simulink library "SG_library"  (R2022b)
settings: Solver=VariableStepAuto  StartTime=0.0  StopTime=10.0  RelTol=1e-3
undefined symbols (not defined in the file or in its folder): a, b, c, ctrl_limit, dfilt, GeneratorType, IO324, IO324_FPGA, IO324_src, IO334, IO334_FPGA, IO334_src, IO397, IO397_FPGA, IO397_src, repelem
libraries: speedgoatlib_hdlCoder_IO3xx x44, $bdroot x14, slrealtimeutilitieslib x9, simulink x8, hdlsllib x6, dsparch4 x2
(part 1 of 3)
settings Model: Creator=mavolery  LastModifiedBy=mavolery

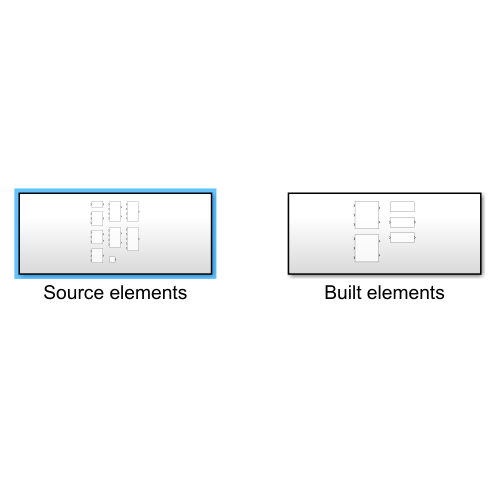
[thumbnail: Simulink's stored preview of the top-level diagram]
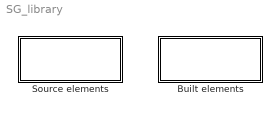
== system SG_library ==
  Built elements : Subsystem
  Source elements : Subsystem

== system SG_library/Built elements ==
  IO324_IO : Subsystem  mask(IO334 IO){ts=-1, adcGain=5.12V, dacGain=5.0V}
      mask prompts: ts "Filters sampling time"; adcGain "ADC range (all channels)"; dacGain "DAC range (all channels)"
      mask help: Links the 16 first physical analog inputs/outputs to the CPU part of the speedgoat.
      mask TypeOptions ts: IO324_SOS/ts
      mask TypeOptions adcGain: IO324_SOS/adcGain
      mask TypeOptions dacGain: IO324_SOS/dacGain
  IO324_SOS : Subsystem  mask(IO334_SOS){sos1=[0 0 0 1 0 0;0 0 0 1 0 0;0 0 0 1 0 0;0 0 0 1 0 0], sos2=[0 0 0 1 0 0;0 0 0 1 0 0;0 0 0 1 0 0;0 0 0 1 0 0], ctrl_limit=-1, ts=-1, channel_in=[1 2], channel_out=1, adcGain=5.12V, dacGain=5.0V}
      mask prompts: sos1 "SOS matrix AI1 -> AO1"; sos2 "SOS matrix AI2 -> AO1"; ctrl_limit "Control output limit [V]"; ts "Filters sampling time"; channel_in "Filter input channels (1-16, 0 for GND)"; channel_out "Filter output channel (1-8)"; adcGain "ADC range (all channels)"; dacGain "DAC range (all channels)"
      mask help: Implements a discrete fixed-point filter by second order sections cascade. SOS matrices are given by tf2sos or zp2sos.
      mask TypeOptions adcGain: IO324_FPGA/adcGain_1 | IO324_FPGA/adcGain_10 | IO324_FPGA/adcGain_11 | IO324_FPGA/adcGain_12 | IO324_FPGA/adcGain_13 | IO324_FPGA/adcGain_14 | IO324_FPGA/adcGain_15 | IO324_FPGA/adcGain_16 | IO324_FPGA/adcGain_17 | IO324_FPGA/adcGain_18 | IO324_FPGA/adcGain_19 | IO324_FPGA/adcGain_2 | IO324_FPGA/adcGain_20 | IO324_FPGA/adcGain_21 | IO324_FPGA/adcGain_22 | IO324_FPGA/adcGain_23 | IO324_FPGA/adcGain_24 | IO324_FPGA/adcGain_25 | IO324_FPGA/adcGain_26 | IO324_FPGA/adcGain_27 | IO324_FPGA/adcGain_28 | IO324_FPGA/adcGain_29 | IO324_FPGA/adcGain_3 | IO324_FPGA/adcGain_30 | IO324_FPGA/adcGain_31 | IO324_FPGA/adcGain_32 | IO324_FPGA/adcGain_4 | IO324_FPGA/adcGain_5 | IO324_FPGA/adcGain_6 | IO324_FPGA/adcGain_7 | IO324_FPGA/adcGain_8 | IO324_FPGA/adcGain_9
      mask TypeOptions dacGain: IO324_FPGA/dacGain_1 | IO324_FPGA/dacGain_2 | IO324_FPGA/dacGain_3 | IO324_FPGA/dacGain_4 | IO324_FPGA/dacGain_5 | IO324_FPGA/dacGain_6 | IO324_FPGA/dacGain_7 | IO324_FPGA/dacGain_8
  IO334_IO : Subsystem  mask(IO334 IO){ts=-1, span=Auto (same as ADC)}
      mask prompts: ts "Sampling time (ADC)"; span "DAC Voltage Range:"
      mask help: Links the 16 first physical analog inputs/outputs to the CPU part of the speedgoat.
      mask TypeOptions ts: IO334_SOS/ts
      mask TypeOptions span: IO334_SOS/span
  IO334_SOS : Subsystem  mask(IO334_SOS){sos1=[0 0 0 1 0 0;0 0 0 1 0 0;0 0 0 1 0 0;0 0 0 1 0 0], sos2=[0 0 0 1 0 0;0 0 0 1 0 0;0 0 0 1 0 0;0 0 0 1 0 0], limit_ctrl=-1, channel_in=[1 2], channel_out=1, ts=-1, span=Auto (same as ADC)}
      mask prompts: sos1 "SOS matrix AI1 -> AO1"; sos2 "SOS matrix AI2 -> AO1"; limit_ctrl "Control output limit [V]"; channel_in "Filter input channels (1-16, 0 for GND)"; channel_out "filtouer output channel (1-16)"; ts "Sampling time (ADC)"; span "DAC Voltage Range:"
      mask help: Implements a discrete fixed-point filter by second order sections cascade. SOS matrices are given by tf2sos or zp2sos.
      mask TypeOptions span: IO334_FPGA/OutputRange
  IO397_IO : Subsystem  mask(IO397 IO){ts=-1, range1=+-10 V, range2=+-10 V, range3=+-10 V, range4=+-10 V, span=+-10 V}
      mask prompts: ts "Sampling time (ADC)"; range1 "Range ADC Channel 1"; range2 "Range ADC Channel 2"; range3 "Range ADC Channel 3"; range4 "Range ADC Channel 4"; span "DAC Voltage Span:"
      mask help: Links the four first physical analog inputs/outputs to the CPU part of the speedgoat.
      mask TypeOptions ts: IO397_SOS/ts
      mask TypeOptions range1: IO397_SOS/range1
      mask TypeOptions range2: IO397_SOS/range2
      mask TypeOptions range3: IO397_SOS/range3
      mask TypeOptions range4: IO397_SOS/range4
      mask TypeOptions span: IO397_SOS/span
      mask DialogControl AnalogInput Prompt: Analog Inputs
      mask DialogControl AnalogOutput Prompt: Analog Output
  IO397_SOS : Subsystem  mask(IO397_SOS){sos1=[1 0 0 1 0 0;1 0 0 1 0 0;1 0 0 1 0 0;1 0 0 1 0 0], sos2=[0 0 0 1 0 0;0 0 0 1 0 0;0 0 0 1 0 0;0 0 0 1 0 0], limit_ctrl=-1, ts=-1, channel_in=[1,2], channel_out=1, range1=+-10 V, range2=+-10 V, range3=+-10 V, range4=+-10 V, span=+-10 V}
      mask prompts: sos1 "SOS matrix AI1 -> AO1"; sos2 "SOS matrix AI2 -> AO1"; limit_ctrl "Control output limit [V]"; ts "Sampling time (ADC)"; channel_in "Filter input channels (1-4, 0 for gnd)"; channel_out "Filter output channel (1-4)"; range1 "Range ADC Channel 1"; range2 "Range ADC Channel 2"; range3 "Range ADC Channel 3"; range4 "Range ADC Channel 4"; span "DAC Voltage Span:"
      mask help: Implements a discrete fixed-point filter by second order sections cascade. SOS matrices are given by tf2sos or zp2sos.
      mask init:
      | assert(all(range1 ~= [1 4 5]), 'ADC1 range must be symetric');
      | assert(all(range2 ~= [1 4 5]), 'ADC2 range must be symetric');
      | assert(all(span ~= [1 2]), 'DAC span must be symetric');
      mask TypeOptions range1: IO397_FPGA/range1
      mask TypeOptions range2: IO397_FPGA/range2
      mask TypeOptions range3: IO397_FPGA/range3
      mask TypeOptions range4: IO397_FPGA/range4
      mask TypeOptions span: IO397_FPGA/span
      mask DialogControl AnalogInput Prompt: Analog Inputs
      mask DialogControl AnalogOutput Prompt: Analog Output
  private : Subsystem

== system SG_library/Source elements ==
  ADC trigger : Subsystem  mask(AI trigger){}
      mask help: Creates a boolean pulse every given cylces. It can be use for ADC acquisition
  Discrete SOS section DFI serial : Subsystem  mask(Discrete fixed-point SOS section){idx=1, OutDataTypeStr=fixdt(1,80,52)}
      mask prompts: idx "Index"; OutDataTypeStr "Accumulator datatype"
      mask help: This is a fixed-point implementation of a biquad filter. Specify the sos [N/2, 6] matrix e.g. given by tf2sos or zpk2sos functions. The first denominator coefficient must always be equal to 1. Index (1 - N/2) parameter specifies which section of the filter is implemented.
      mask TypeOptions OutDataTypeStr: Signal Specification/OutDataTypeStr
  Discrete SOS serial : Subsystem  mask(Discrete fixed-point second order sections filter){OutDataTypeStr=fixdt(1,80,52)}
      mask prompts: OutDataTypeStr "Accumulator datatype"
      mask help: This is a SOS implemetation of order 8 (4 sections). Specify the sos [n/2, 6] matrix e.g. given by tf2sos function. The first denominator coefficient must always be equal to 1.
      mask TypeOptions OutDataTypeStr:
      | Discrete SOS
      | section DFI serial/OutDataTypeStr
  Generator : Subsystem  mask(Generator){duration=10, rms=1, f1=50, f2=500, gen_type=GeneratorType.rand_white, ts=-1}
      mask prompts: duration "Duration [s]"; rms "RMS value"; f1 "Start frequency [Hz] (sweep only)"; f2 "Stop frequency [Hz] (sweep only)"; gen_type "Type (GeneratorType)"; ts "Sampling time [s]"
      mask help: Runs different types of generators for a given duration. Generator can be triggered, canceled and manually enabled.
  Linear Chirp : Subsystem  mask{f1=10, f2=50, t_sweep=2.64, ts=-1}
      mask prompts: f1 "Start frequency"; f2 "End frequency"; t_sweep "Sweep time"; ts "Sample time"
  Logarithmic Chirp : Subsystem  mask{f1=10, f2=50, t_sweep=2.64, ts=-1}
      mask prompts: f1 "Start frequency"; f2 "End frequency"; t_sweep "Sweep time"; ts "Sample time"
  Random source : Subsystem  mask(Random source){mean=0, stdev=1, seed=0, SampleTime=0.0001}
      mask prompts: stdev "Standard deviation"; SampleTime "Sample time"
      mask help: Creates some random signal, limited in frequency at Fs/4
  SOS filter : Subsystem  mask(SOS filter){sos1=[0 0 0 1 0 0;0 0 0 1 0 0;0 0 0 1 0 0;0 0 0 1 0 0], sos2=[0 0 0 1 0 0;0 0 0 1 0 0;0 0 0 1 0 0;0 0 0 1 0 0], limit_ctrl=10, ts=-1}
      mask prompts: sos1 "SOS matrix AI1 -> AO1"; sos2 "SOS matrix AI2 -> AO1"; limit_ctrl "Control output limit [V]"; ts "Filter sampling time [s]"
      mask help: Implements a discrete fixed-point filter by second order sections cascade. SOS matrices are given by tf2sos or zp2sos.
  Triggered Pulse : Subsystem  mask(Triggered Pulse){}
      mask help: Generates a single pulse of N samples length

== system SG_library/Built elements/IO324_IO ==
  AO : Inport
  Constant : Constant  Value=false  SampleTime=-1
  Constant1 : Constant  Value=false  SampleTime=-1
  IO324_SOS : $bdroot/Built elements/IO324_SOS  sos1=[0 0 0 1 0 0;0 0 0 1 0 0;0 0 0 1 0 0;0 0 0 1 0 0]  sos2=[0 0 0 1 0 0;0 0 0 1 0 0;0 0 0 1 0 0;0 0 0 1 0 0]  ctrl_limit=-1  ts=ts  channel_in=[1 2]  channel_out=1  adcGain=5.12V  dacGain=5.0V
      settings: LibrarySourceBlock=libpanache/IO324_SOS
  Rate Transition : RateTransition  OutPortSampleTime=ts
  Terminator : Terminator
  Terminator1 : Terminator
  AI : Outport  VectorParamsAs1DForOutWhenUnconnected=off
  wires:
  Constant/1 -> IO324_SOS/2
  AO/1 -> IO324_SOS/1
  IO324_SOS/1 -> Rate Transition/1
  Rate Transition/1 -> AI/1
  IO324_SOS/2 -> Terminator/1
  Constant1/1 -> IO324_SOS/3
  IO324_SOS/3 -> Terminator1/1

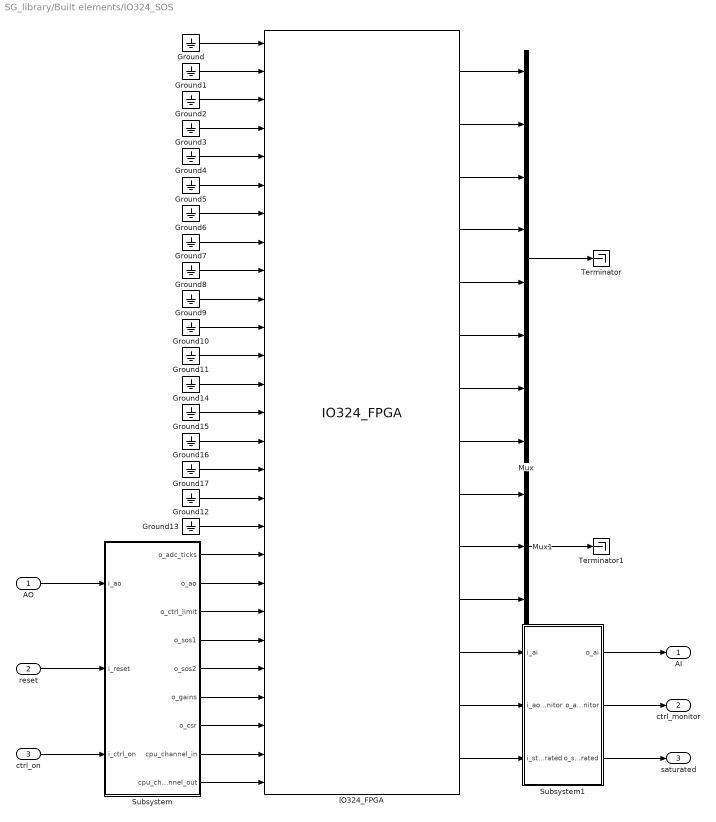
== system SG_library/Built elements/IO324_SOS ==
  AO : Inport  PortDimensions=8
  reset : Inport  Port=2  OutDataTypeStr=boolean  PortDimensions=1
  ctrl_on : Inport  Port=3  OutDataTypeStr=boolean  PortDimensions=1
  Ground{,1..17} (18 alike) : Ground
  IO324_FPGA : $bdroot/Built elements/private/IO324_FPGA  module_id=1  slot=-1  ts=-1  adcGain_1=5.12V  adcActiv_1=on  adcDiffSelect_1=off  adcGain_2=5.12V  adcActiv_2=on  adcDiffSelect_2=off  adcGain_3=5.12V  adcActiv_3=off  adcDiffSelect_3=off  adcGain_4=5.12V  adcActiv_4=off  adcDiffSelect_4=off  adcGain_5=5.12V  adcActiv_5=off  adcDiffSelect_5=off  adcGain_6=5.12V  adcActiv_6=off  adcDiffSelect_6=off  adcGain_7=5.12V  adcActiv_7=off  adcDiffSelect_7=off  adcGain_8=5.12V  adcActiv_8=off  adcDiffSelect_8=off  adcGain_9=5.12V  adcActiv_9=on  adcDiffSelect_9=off  adcGain_10=5.12V  adcActiv_10=on  adcDiffSelect_10=off  adcGain_11=5.12V  adcActiv_11=off  adcDiffSelect_11=off  adcGain_12=5.12V  adcActiv_12=off  adcDiffSelect_12=off  adcGain_13=5.12V  adcActiv_13=off  adcDiffSelect_13=off  adcGain_14=5.12V  adcActiv_14=off  adcDiffSelect_14=off  adcGain_15=5.12V  adcActiv_15=off  adcDiffSelect_15=off  adcGain_16=5.12V  adcActiv_16=off  adcDiffSelect_16=off  adcGain_17=5.12V  adcActiv_17=on  adcDiffSelect_17=off  adcGain_18=5.12V  adcActiv_18=on  adcDiffSelect_18=off  adcGain_19=5.12V  adcActiv_19=off  adcDiffSelect_19=off  adcGain_20=5.12V  adcActiv_20=off  adcDiffSelect_20=off  adcGain_21=5.12V  adcActiv_21=off  adcDiffSelect_21=off  adcGain_22=5.12V  adcActiv_22=off  adcDiffSelect_22=off  adcGain_23=5.12V  adcActiv_23=off  adcDiffSelect_23=off  adcGain_24=5.12V  adcActiv_24=off  adcDiffSelect_24=off  adcGain_25=5.12V  adcActiv_25=on  adcDiffSelect_25=off  adcGain_26=5.12V  adcActiv_26=on  adcDiffSelect_26=off  adcGain_27=5.12V  adcActiv_27=off  adcDiffSelect_27=off  adcGain_28=5.12V  adcActiv_28=off  adcDiffSelect_28=off  adcGain_29=5.12V  adcActiv_29=off  adcDiffSelect_29=off  adcGain_30=5.12V  adcActiv_30=off  adcDiffSelect_30=off  adcGain_31=5.12V  adcActiv_31=off  adcDiffSelect_31=off  adcGain_32=5.12V  adcActiv_32=off  adcDiffSelect_32=off  dacGain_1=5.0V  dacActiv_1=on  dacGain_2=5.0V  dacActiv_2=on  dacGain_3=5.0V  dacActiv_3=on  dacGain_4=5.0V  dacActiv_4=on  dacGain_5=5.0V  dacActiv_5=on  dacGain_6=5.0V  dacActiv_6=on  dacGain_7=5.0V  dacActiv_7=on  dacGain_8=5.0V  dacActiv_8=on  fpga_sync_mode=on  reset_mode=on  reset_mode_stop=on  FpgaFreq=100
      settings: LibrarySourceBlock=libpanache/private/IO324_FPGA
  Mux : Mux  Inputs=8
  Mux1 : Mux  Inputs=3
  Subsystem : Subsystem
  Subsystem1 : Subsystem
  Terminator : Terminator
  Terminator1 : Terminator
  AI : Outport  VectorParamsAs1DForOutWhenUnconnected=off
  ctrl_monitor : Outport  Port=2  VectorParamsAs1DForOutWhenUnconnected=off
  saturated : Outport  Port=3
  wires:
  Ground/1 -> IO324_FPGA/1
  Ground1/1 -> IO324_FPGA/2
  Ground2/1 -> IO324_FPGA/3
  Ground3/1 -> IO324_FPGA/4
  Ground4/1 -> IO324_FPGA/5
  Ground7/1 -> IO324_FPGA/8
  Ground6/1 -> IO324_FPGA/7
  Ground5/1 -> IO324_FPGA/6
  Ground9/1 -> IO324_FPGA/10
  Ground10/1 -> IO324_FPGA/11
  Ground8/1 -> IO324_FPGA/9
  Ground11/1 -> IO324_FPGA/12
  AO/1 -> Subsystem/1(i_ao)
  ctrl_on/1 -> Subsystem/3(i_ctrl_on)
  reset/1 -> Subsystem/2(i_reset)
  Subsystem1/1(o_ai) -> AI/1
  Subsystem1/2(o_ao_monitor) -> ctrl_monitor/1
  IO324_FPGA/12 -> Subsystem1/1(i_ai)
  IO324_FPGA/13 -> Subsystem1/2(i_ao_monitor)
  Subsystem/7(o_csr) -> IO324_FPGA/25
  Subsystem/2(o_ao) -> IO324_FPGA/20
  Subsystem/3(o_ctrl_limit) -> IO324_FPGA/21
  Subsystem/4(o_sos1) -> IO324_FPGA/22
  Subsystem/5(o_sos2) -> IO324_FPGA/23
  Subsystem/6(o_gains) -> IO324_FPGA/24
  Subsystem/1(o_adc_ticks) -> IO324_FPGA/19
  Ground16/1 -> IO324_FPGA/15
  Ground12/1 -> IO324_FPGA/17
  Ground17/1 -> IO324_FPGA/16
  Ground15/1 -> IO324_FPGA/14
  Ground14/1 -> IO324_FPGA/13
  Ground13/1 -> IO324_FPGA/18
  IO324_FPGA/1 -> Mux/1
  IO324_FPGA/2 -> Mux/2
  IO324_FPGA/3 -> Mux/3
  IO324_FPGA/4 -> Mux/4
  IO324_FPGA/5 -> Mux/5
  IO324_FPGA/6 -> Mux/6
  IO324_FPGA/7 -> Mux/7
  IO324_FPGA/8 -> Mux/8
  Mux/1 -> Terminator/1
  IO324_FPGA/9 -> Mux1/1
  IO324_FPGA/10 -> Mux1/2
  IO324_FPGA/11 -> Mux1/3
  IO324_FPGA/14 -> Subsystem1/3(i_staurated)
  Subsystem1/3(o_saturated) -> saturated/1
  Subsystem/8(cpu_channel_in) -> IO324_FPGA/26
  Subsystem/9(cpu_channel_out) -> IO324_FPGA/27
  Mux1/1 -> Terminator1/1

== system SG_library/Built elements/IO334_IO ==
  AO : Inport
  Constant : Constant  Value=false  SampleTime=-1
  IO334_SOS : $bdroot/Built elements/IO334_SOS  sos1=[0 0 0 1 0 0;0 0 0 1 0 0;0 0 0 1 0 0;0 0 0 1 0 0]  sos2=[0 0 0 1 0 0;0 0 0 1 0 0;0 0 0 1 0 0;0 0 0 1 0 0]  limit_ctrl=-1  channel_in=[1 2]  channel_out=1  ts=ts  span=Auto (same as ADC)
      settings: LibrarySourceBlock=SG_library_TRASH/Built elements/IO334_SOS
  Rate Transition : RateTransition  OutPortSampleTime=ts
  Terminator : Terminator
  Terminator1 : Terminator
  AI : Outport  VectorParamsAs1DForOutWhenUnconnected=off
  wires:
  Constant/1 -> IO334_SOS/3, IO334_SOS/2
  AO/1 -> IO334_SOS/1
  IO334_SOS/1 -> Rate Transition/1
  Rate Transition/1 -> AI/1
  IO334_SOS/2 -> Terminator/1
  IO334_SOS/3 -> Terminator1/1

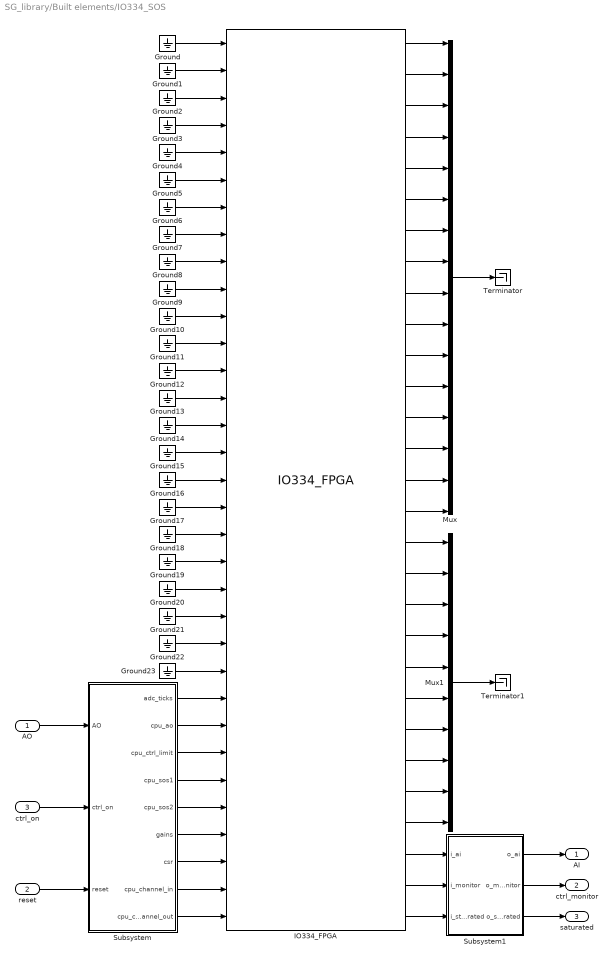
== system SG_library/Built elements/IO334_SOS ==
  AO : Inport
  reset : Inport  Port=2
  ctrl_on : Inport  Port=3
  Ground{,1..23} (24 alike) : Ground
  IO334_FPGA : $bdroot/Built elements/private/IO334_FPGA  module_id=1  slot=-1  ts=-1  OutputRange=Auto (same as ADC)  fpga_sync_mode=on  reset_mode=on  reset_mode_stop=on  FpgaFreq=100
      settings: LibrarySourceBlock=SG_library_TRASH/Built elements/private/IO334_FPGA
  Mux : Mux  Inputs=16
  Mux1 : Mux  Inputs=10
  Subsystem : Subsystem
  Subsystem1 : Subsystem
  Terminator : Terminator
  Terminator1 : Terminator
  AI : Outport  VectorParamsAs1DForOutWhenUnconnected=off
  ctrl_monitor : Outport  Port=2  VectorParamsAs1DForOutWhenUnconnected=off
  saturated : Outport  Port=3
  wires:
  IO334_FPGA/1 -> Mux/1
  IO334_FPGA/2 -> Mux/2
  IO334_FPGA/3 -> Mux/3
  IO334_FPGA/4 -> Mux/4
  IO334_FPGA/5 -> Mux/5
  IO334_FPGA/6 -> Mux/6
  IO334_FPGA/7 -> Mux/7
  IO334_FPGA/8 -> Mux/8
  IO334_FPGA/9 -> Mux/9
  IO334_FPGA/10 -> Mux/10
  IO334_FPGA/11 -> Mux/11
  IO334_FPGA/12 -> Mux/12
  IO334_FPGA/13 -> Mux/13
  IO334_FPGA/14 -> Mux/14
  IO334_FPGA/15 -> Mux/15
  IO334_FPGA/16 -> Mux/16
  Mux/1 -> Terminator/1
  IO334_FPGA/17 -> Mux1/1
  IO334_FPGA/18 -> Mux1/2
  IO334_FPGA/19 -> Mux1/3
  IO334_FPGA/20 -> Mux1/4
  IO334_FPGA/21 -> Mux1/5
  IO334_FPGA/22 -> Mux1/6
  IO334_FPGA/23 -> Mux1/7
  IO334_FPGA/24 -> Mux1/8
  IO334_FPGA/25 -> Mux1/9
  IO334_FPGA/26 -> Mux1/10
  Mux1/1 -> Terminator1/1
  Ground/1 -> IO334_FPGA/1
  Ground1/1 -> IO334_FPGA/2
  Ground2/1 -> IO334_FPGA/3
  Ground3/1 -> IO334_FPGA/4
  Ground5/1 -> IO334_FPGA/6
  Ground6/1 -> IO334_FPGA/7
  Ground7/1 -> IO334_FPGA/8
  Ground4/1 -> IO334_FPGA/5
  Ground10/1 -> IO334_FPGA/11
  Ground13/1 -> IO334_FPGA/14
  Ground12/1 -> IO334_FPGA/13
  Ground14/1 -> IO334_FPGA/15
  Ground15/1 -> IO334_FPGA/16
  Ground9/1 -> IO334_FPGA/10
  Ground11/1 -> IO334_FPGA/12
  Ground8/1 -> IO334_FPGA/9
  Ground18/1 -> IO334_FPGA/19
  Ground21/1 -> IO334_FPGA/22
  Ground20/1 -> IO334_FPGA/21
  Ground22/1 -> IO334_FPGA/23
  Ground23/1 -> IO334_FPGA/24
  Ground17/1 -> IO334_FPGA/18
  Ground19/1 -> IO334_FPGA/20
  Ground16/1 -> IO334_FPGA/17
  IO334_FPGA/27 -> Subsystem1/1(i_ai)
  IO334_FPGA/28 -> Subsystem1/2(i_monitor)
  Subsystem1/1(o_ai) -> AI/1
  Subsystem1/2(o_monitor) -> ctrl_monitor/1
  AO/1 -> Subsystem/1(AO)
  Subsystem/1(adc_ticks) -> IO334_FPGA/25
  Subsystem/2(cpu_ao) -> IO334_FPGA/26
  Subsystem/3(cpu_ctrl_limit) -> IO334_FPGA/27
  Subsystem/4(cpu_sos1) -> IO334_FPGA/28
  Subsystem/5(cpu_sos2) -> IO334_FPGA/29
  Subsystem/6(gains) -> IO334_FPGA/30
  Subsystem/7(csr) -> IO334_FPGA/31
  reset/1 -> Subsystem/3(reset)
  ctrl_on/1 -> Subsystem/2(ctrl_on)
  Subsystem/8(cpu_channel_in) -> IO334_FPGA/32
  Subsystem/9(cpu_channel_out) -> IO334_FPGA/33
  IO334_FPGA/29 -> Subsystem1/3(i_staurated)
  Subsystem1/3(o_saturated) -> saturated/1

== system SG_library/Built elements/IO397_IO ==
  AO : Inport
  Constant : Constant  Value=false  SampleTime=-1
  IO397_SOS : $bdroot/Built elements/IO397_SOS  sos1=[1 0 0 1 0 0;1 0 0 1 0 0;1 0 0 1 0 0;1 0 0 1 0 0]  sos2=[0 0 0 1 0 0;0 0 0 1 0 0;0 0 0 1 0 0;0 0 0 1 0 0]  limit_ctrl=-1  ts=ts  channel_in=[1,2]  channel_out=1  range1=+-10 V  range2=+-10 V  range3=+-10 V  range4=+-10 V  span=+-10 V
      settings: LibrarySourceBlock=SG_library_TRASH/Built elements/IO397_SOS
  Rate Transition : RateTransition  OutPortSampleTime=ts
  Terminator : Terminator
  Terminator1 : Terminator
  AI : Outport  VectorParamsAs1DForOutWhenUnconnected=off
  wires:
  AO/1 -> IO397_SOS/1
  IO397_SOS/1 -> Rate Transition/1
  Constant/1 -> IO397_SOS/2, IO397_SOS/3
  Rate Transition/1 -> AI/1
  IO397_SOS/2 -> Terminator/1
  IO397_SOS/3 -> Terminator1/1

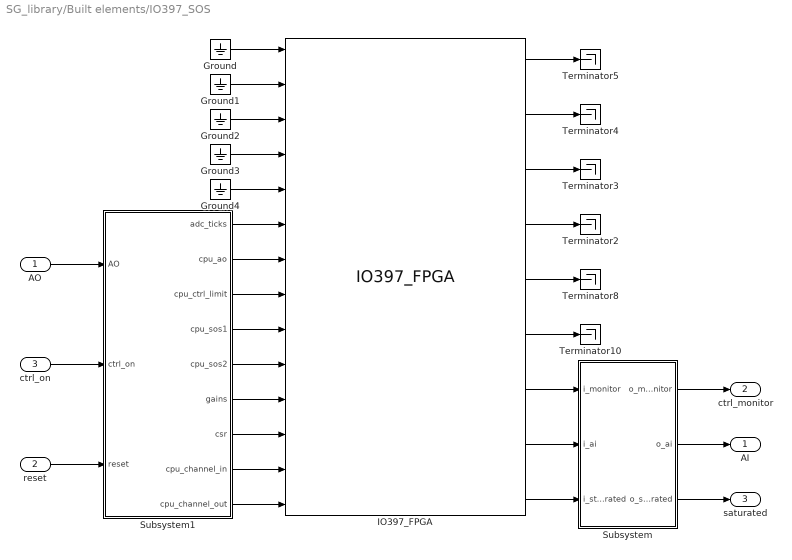
== system SG_library/Built elements/IO397_SOS ==
  AO : Inport
  reset : Inport  Port=2
  ctrl_on : Inport  Port=3
  Ground{,1..4} (5 alike) : Ground
  IO397_FPGA : $bdroot/Built elements/private/IO397_FPGA  module_id=1  slot=-1  ts=-1  range1=+-10 V  range2=+-10 V  range3=+-10 V  range4=+-10 V  span=+-10 V  fpga_sync_mode=on  reset_mode=on  reset_mode_stop=on  FpgaFreq=100
      settings: LibrarySourceBlock=SG_library_TRASH/Built elements/private/IO397_FPGA
  Subsystem : Subsystem
  Subsystem1 : Subsystem
  Terminator{2..5,8,10} (6 alike) : Terminator
  AI : Outport  VectorParamsAs1DForOutWhenUnconnected=off
  ctrl_monitor : Outport  Port=2  VectorParamsAs1DForOutWhenUnconnected=off
  saturated : Outport  Port=3
  wires:
  IO397_FPGA/2 -> Terminator4/1
  IO397_FPGA/6 -> Terminator10/1
  IO397_FPGA/5 -> Terminator8/1
  IO397_FPGA/4 -> Terminator2/1
  IO397_FPGA/3 -> Terminator3/1
  IO397_FPGA/1 -> Terminator5/1
  Ground/1 -> IO397_FPGA/1
  Ground1/1 -> IO397_FPGA/2
  Ground2/1 -> IO397_FPGA/3
  Ground3/1 -> IO397_FPGA/4
  Ground4/1 -> IO397_FPGA/5
  IO397_FPGA/7 -> Subsystem/1(i_monitor)
  IO397_FPGA/8 -> Subsystem/2(i_ai)
  Subsystem/1(o_monitor) -> ctrl_monitor/1
  Subsystem/2(o_ai) -> AI/1
  AO/1 -> Subsystem1/1(AO)
  ctrl_on/1 -> Subsystem1/2(ctrl_on)
  reset/1 -> Subsystem1/3(reset)
  Subsystem1/1(adc_ticks) -> IO397_FPGA/6
  Subsystem1/2(cpu_ao) -> IO397_FPGA/7
  Subsystem1/3(cpu_ctrl_limit) -> IO397_FPGA/8
  Subsystem1/4(cpu_sos1) -> IO397_FPGA/9
  Subsystem1/5(cpu_sos2) -> IO397_FPGA/10
  Subsystem1/6(gains) -> IO397_FPGA/11
  Subsystem1/7(csr) -> IO397_FPGA/12
  Subsystem1/8(cpu_channel_in) -> IO397_FPGA/13
  Subsystem1/9(cpu_channel_out) -> IO397_FPGA/14
  IO397_FPGA/9 -> Subsystem/3(i_staurated)
  Subsystem/3(o_saturated) -> saturated/1

== system SG_library/Built elements/private ==
  IO324_FPGA : Subsystem  mask(Speedgoat IO324-200k Interface Block){module_id=1, slot=-1, ts=-1, adcGain_1=10.24V, adcActiv_1=on, adcDiffSelect_1=off, adcGain_2=10.24V, adcActiv_2=on, adcDiffSelect_2=off, adcGain_3=10.24V, adcActiv_3=on, adcDiffSelect_3=off, adcGain_4=10.24V, adcActiv_4=on, adcDiffSelect_4=off, adcGain_5=10.24V, adcActiv_5=on, adcDiffSelect_5=off, adcGain_6=10.24V, adcActiv_6=on, adcDiffSelect_6=off, adcGain_7=10.24V, adcActiv_7=on, adcDiffSelect_7=off, adcGain_8=10.24V, adcActiv_8=on, adcDiffSelect_8=off, adcGain_9=10.24V, adcActiv_9=on, adcDiffSelect_9=off, adcGain_10=10.24V, adcActiv_10=on, adcDiffSelect_10=off, adcGain_11=10.24V, adcActiv_11=on, adcDiffSelect_11=off, adcGain_12=10.24V, adcActiv_12=on, adcDiffSelect_12=off, adcGain_13=10.24V, adcActiv_13=on, adcDiffSelect_13=off, adcGain_14=10.24V, adcActiv_14=on, adcDiffSelect_14=off, adcGain_15=10.24V, adcActiv_15=on, adcDiffSelect_15=off, adcGain_16=10.24V, adcActiv_16=on, adcDiffSelect_16=off, adcGain_17=10.24V, adcActiv_17=off, adcDiffSelect_17=off, adcGain_18=10.24V, adcActiv_18=off, adcDiffSelect_18=off, adcGain_19=10.24V, adcActiv_19=off, adcDiffSelect_19=off, adcGain_20=10.24V, adcActiv_20=off, adcDiffSelect_20=off, adcGain_21=10.24V, adcActiv_21=off, adcDiffSelect_21=off, adcGain_22=10.24V, adcActiv_22=off, adcDiffSelect_22=off, adcGain_23=10.24V, adcActiv_23=off, adcDiffSelect_23=off, adcGain_24=10.24V, adcActiv_24=off, adcDiffSelect_24=off, adcGain_25=10.24V, adcActiv_25=off, adcDiffSelect_25=off, adcGain_26=10.24V, adcActiv_26=off, adcDiffSelect_26=off, adcGain_27=10.24V, adcActiv_27=off, adcDiffSelect_27=off, adcGain_28=10.24V, adcActiv_28=off, adcDiffSelect_28=off, adcGain_29=10.24V, adcActiv_29=off, adcDiffSelect_29=off, adcGain_30=10.24V, adcActiv_30=off, adcDiffSelect_30=off, adcGain_31=10.24V, adcActiv_31=off, adcDiffSelect_31=off, adcGain_32=10.24V, adcActiv_32=off, adcDiffSelect_32=off, dacGain_1=10.0V, dacActiv_1=on, dacGain_2=10.0V, dacActiv_2=on, dacGain_3=10.0V, dacActiv_3=on, dacGain_4=10.0V, dacActiv_4=on, dacGain_5=10.0V, dacActiv_5=on, dacGain_6=10.0V, dacActiv_6=on, dacGain_7=10.0V, dacActiv_7=on, dacGain_8=10.0V, dacActiv_8=on, fpga_sync_mode=on, reset_mode=on, reset_mode_stop=on, FpgaFreq=100}
      mask prompts: module_id "FPGA Module Identifier:"; slot "PCI slot (-1: autosearch):"; ts "Sample time:"; adcGain_1 "ADC Ch 01 Range"; adcActiv_1 "Activ"; adcDiffSelect_1 "Differential with Ch 02"; adcGain_2 "ADC Ch 02 Range"; adcActiv_2 "Activ"; adcDiffSelect_2 "Differential with Ch 01"; adcGain_3 "ADC Ch 03 Range"; adcActiv_3 "Activ"; adcDiffSelect_3 "Differential with Ch 04"; adcGain_4 "ADC Ch 04 Range"; adcActiv_4 "Activ"; adcDiffSelect_4 "Differential with Ch 03"; adcGain_5 "ADC Ch 05 Range"; adcActiv_5 "Activ"; adcDiffSelect_5 "Differential with Ch 06"; adcGain_6 "ADC Ch 06 Range"; adcActiv_6 "Activ"; adcDiffSelect_6 "Differential with Ch 05"; adcGain_7 "ADC Ch 07 Range"; adcActiv_7 "Activ"; adcDiffSelect_7 "Differential with Ch 08"; adcGain_8 "ADC Ch 08 Range"; adcActiv_8 "Activ"; adcDiffSelect_8 "Differential with Ch 07"; adcGain_9 "ADC Ch 09 Range"; adcActiv_9 "Activ"; adcDiffSelect_9 "Differential with Ch 10"; adcGain_10 "ADC Ch 10 Range"; adcActiv_10 "Activ"; adcDiffSelect_10 "Differential with Ch 09"; adcGain_11 "ADC Ch 11 Range"; adcActiv_11 "Activ"; adcDiffSelect_11 "Differential with Ch 12"; adcGain_12 "ADC Ch 12 Range"; adcActiv_12 "Activ"; adcDiffSelect_12 "Differential with Ch 11"; adcGain_13 "ADC Ch 13 Range"; adcActiv_13 "Activ"; adcDiffSelect_13 "Differential with Ch 14"; adcGain_14 "ADC Ch 14 Range"; adcActiv_14 "Activ"; adcDiffSelect_14 "Differential with Ch 13"; adcGain_15 "ADC Ch 15 Range"; adcActiv_15 "Activ"; adcDiffSelect_15 "Differential with Ch 16"; adcGain_16 "ADC Ch 16 Range"; adcActiv_16 "Activ"; adcDiffSelect_16 "Differential with Ch 15"; adcGain_17 "ADC Ch 17 Range"; adcActiv_17 "Activ"; adcDiffSelect_17 "Differential with Ch 18"; adcGain_18 "ADC Ch 18 Range"; adcActiv_18 "Activ"; adcDiffSelect_18 "Differential with Ch 17"; adcGain_19 "ADC Ch 19 Range"; adcActiv_19 "Activ"; adcDiffSelect_19 "Differential with Ch 20"; adcGain_20 "ADC Ch 20 Range"; adcActiv_20 "Activ"; adcDiffSelect_20 "Differential with Ch 19"; adcGain_21 "ADC Ch 21 Range"; adcActiv_21 "Activ"; adcDiffSelect_21 "Differential with Ch 22"; adcGain_22 "ADC Ch 22 Range"; adcActiv_22 "Activ"; adcDiffSelect_22 "Differential with Ch 21"; adcGain_23 "ADC Ch 23 Range"; adcActiv_23 "Activ"; adcDiffSelect_23 "Differential with Ch 24"; adcGain_24 "ADC Ch 24 Range"; adcActiv_24 "Activ"; adcDiffSelect_24 "Differential with Ch 23"; adcGain_25 "ADC Ch 25 Range"; adcActiv_25 "Activ"; adcDiffSelect_25 "Differential with Ch 26"; adcGain_26 "ADC Ch 26 Range"; adcActiv_26 "Activ"; adcDiffSelect_26 "Differential with Ch 25"; adcGain_27 "ADC Ch 27 Range"; adcActiv_27 "Activ"; adcDiffSelect_27 "Differential with Ch 28"; adcGain_28 "ADC Ch 28 Range"; adcActiv_28 "Activ"; adcDiffSelect_28 "Differential with Ch 27"; adcGain_29 "ADC Ch 29 Range"; adcActiv_29 "Activ"; adcDiffSelect_29 "Differential with Ch 30"; adcGain_30 "ADC Ch 30 Range"; adcActiv_30 "Activ"; adcDiffSelect_30 "Differential with Ch 29"; adcGain_31 "ADC Ch 31 Range"; adcActiv_31 "Activ"; adcDiffSelect_31 "Differential with Ch 32"; adcGain_32 "ADC Ch 32 Range"; adcActiv_32 "Activ"; adcDiffSelect_32 "Differential with Ch 31"; dacGain_1 "DAC Ch 01 Range"; dacActiv_1 "Activ"; dacGain_2 "DAC Ch 02 Range"; dacActiv_2 "Activ"; dacGain_3 "DAC Ch 03 Range"; dacActiv_3 "Activ"; dacGain_4 "DAC Ch 04 Range"; dacActiv_4 "Activ"; dacGain_5 "DAC Ch 05 Range"; dacActiv_5 "Activ"; dacGain_6 "DAC Ch 06 Range"; dacActiv_6 "Activ"; dacGain_7 "DAC Ch 07 Range"; dacActiv_7 "Activ"; dacGain_8 "DAC Ch 08 Range"; dacActiv_8 "Activ"; fpga_sync_mode "Run FPGA only when target application runs"; reset_mode "Reset FPGA states on start"; reset_mode_stop "Reset FPGA states on stop"; FpgaFreq "FPGA Frequency [MHz]"
      mask help: Simulink Real-Time Interface Block for Speedgoat IO324-200k.
      mask init:
      | hdlslrt.backend.mfpgaparameters;
      mask Help: eval('speedgoatdoc_hdlc')
      mask TypeOptions adcGain_1: IO324 ADC Setup/adcGain_1
      mask TypeOptions adcActiv_1: IO324 ADC Setup/adcActiv_1
      mask TypeOptions adcDiffSelect_1: IO324 ADC Setup/adcDiffSelect_1
      mask TypeOptions adcGain_2: IO324 ADC Setup/adcGain_2
      mask TypeOptions adcActiv_2: IO324 ADC Setup/adcActiv_2
      mask TypeOptions adcDiffSelect_2: IO324 ADC Setup/adcDiffSelect_2
      mask TypeOptions adcGain_3: IO324 ADC Setup/adcGain_3
      mask TypeOptions adcActiv_3: IO324 ADC Setup/adcActiv_3
      mask TypeOptions adcDiffSelect_3: IO324 ADC Setup/adcDiffSelect_3
      mask TypeOptions adcGain_4: IO324 ADC Setup/adcGain_4
      mask TypeOptions adcActiv_4: IO324 ADC Setup/adcActiv_4
      mask TypeOptions adcDiffSelect_4: IO324 ADC Setup/adcDiffSelect_4
      mask TypeOptions adcGain_5: IO324 ADC Setup/adcGain_5
      mask TypeOptions adcActiv_5: IO324 ADC Setup/adcActiv_5
      mask TypeOptions adcDiffSelect_5: IO324 ADC Setup/adcDiffSelect_5
      mask TypeOptions adcGain_6: IO324 ADC Setup/adcGain_6
      mask TypeOptions adcActiv_6: IO324 ADC Setup/adcActiv_6
      mask TypeOptions adcDiffSelect_6: IO324 ADC Setup/adcDiffSelect_6
      mask TypeOptions adcGain_7: IO324 ADC Setup/adcGain_7
      mask TypeOptions adcActiv_7: IO324 ADC Setup/adcActiv_7
      mask TypeOptions adcDiffSelect_7: IO324 ADC Setup/adcDiffSelect_7
      mask TypeOptions adcGain_8: IO324 ADC Setup/adcGain_8
      mask TypeOptions adcActiv_8: IO324 ADC Setup/adcActiv_8
      mask TypeOptions adcDiffSelect_8: IO324 ADC Setup/adcDiffSelect_8
      mask TypeOptions adcGain_9: IO324 ADC Setup/adcGain_9
      mask TypeOptions adcActiv_9: IO324 ADC Setup/adcActiv_9
      mask TypeOptions adcDiffSelect_9: IO324 ADC Setup/adcDiffSelect_9
      mask TypeOptions adcGain_10: IO324 ADC Setup/adcGain_10
      mask TypeOptions adcActiv_10: IO324 ADC Setup/adcActiv_10
      mask TypeOptions adcDiffSelect_10: IO324 ADC Setup/adcDiffSelect_10
      mask TypeOptions adcGain_11: IO324 ADC Setup/adcGain_11
      mask TypeOptions adcActiv_11: IO324 ADC Setup/adcActiv_11
      mask TypeOptions adcDiffSelect_11: IO324 ADC Setup/adcDiffSelect_11
      mask TypeOptions adcGain_12: IO324 ADC Setup/adcGain_12
      mask TypeOptions adcActiv_12: IO324 ADC Setup/adcActiv_12
      mask TypeOptions adcDiffSelect_12: IO324 ADC Setup/adcDiffSelect_12
      mask TypeOptions adcGain_13: IO324 ADC Setup/adcGain_13
      mask TypeOptions adcActiv_13: IO324 ADC Setup/adcActiv_13
      mask TypeOptions adcDiffSelect_13: IO324 ADC Setup/adcDiffSelect_13
      mask TypeOptions adcGain_14: IO324 ADC Setup/adcGain_14
      mask TypeOptions adcActiv_14: IO324 ADC Setup/adcActiv_14
      mask TypeOptions adcDiffSelect_14: IO324 ADC Setup/adcDiffSelect_14
      mask TypeOptions adcGain_15: IO324 ADC Setup/adcGain_15
      mask TypeOptions adcActiv_15: IO324 ADC Setup/adcActiv_15
      mask TypeOptions adcDiffSelect_15: IO324 ADC Setup/adcDiffSelect_15
      mask TypeOptions adcGain_16: IO324 ADC Setup/adcGain_16
      mask TypeOptions adcActiv_16: IO324 ADC Setup/adcActiv_16
      mask TypeOptions adcDiffSelect_16: IO324 ADC Setup/adcDiffSelect_16
      mask TypeOptions adcGain_17: IO324 ADC Setup/adcGain_17
      mask TypeOptions adcActiv_17: IO324 ADC Setup/adcActiv_17
      mask TypeOptions adcDiffSelect_17: IO324 ADC Setup/adcDiffSelect_17
      mask TypeOptions adcGain_18: IO324 ADC Setup/adcGain_18
      mask TypeOptions adcActiv_18: IO324 ADC Setup/adcActiv_18
      mask TypeOptions adcDiffSelect_18: IO324 ADC Setup/adcDiffSelect_18
      mask TypeOptions adcGain_19: IO324 ADC Setup/adcGain_19
      mask TypeOptions adcActiv_19: IO324 ADC Setup/adcActiv_19
      mask TypeOptions adcDiffSelect_19: IO324 ADC Setup/adcDiffSelect_19
      mask TypeOptions adcGain_20: IO324 ADC Setup/adcGain_20
      mask TypeOptions adcActiv_20: IO324 ADC Setup/adcActiv_20
      mask TypeOptions adcDiffSelect_20: IO324 ADC Setup/adcDiffSelect_20
      mask TypeOptions adcGain_21: IO324 ADC Setup/adcGain_21
      mask TypeOptions adcActiv_21: IO324 ADC Setup/adcActiv_21
      mask TypeOptions adcDiffSelect_21: IO324 ADC Setup/adcDiffSelect_21
      mask TypeOptions adcGain_22: IO324 ADC Setup/adcGain_22
      mask TypeOptions adcActiv_22: IO324 ADC Setup/adcActiv_22
      mask TypeOptions adcDiffSelect_22: IO324 ADC Setup/adcDiffSelect_22
      mask TypeOptions adcGain_23: IO324 ADC Setup/adcGain_23
      mask TypeOptions adcActiv_23: IO324 ADC Setup/adcActiv_23
      mask TypeOptions adcDiffSelect_23: IO324 ADC Setup/adcDiffSelect_23
      mask TypeOptions adcGain_24: IO324 ADC Setup/adcGain_24
      mask TypeOptions adcActiv_24: IO324 ADC Setup/adcActiv_24
      mask TypeOptions adcDiffSelect_24: IO324 ADC Setup/adcDiffSelect_24
      mask TypeOptions adcGain_25: IO324 ADC Setup/adcGain_25
      mask TypeOptions adcActiv_25: IO324 ADC Setup/adcActiv_25
      mask TypeOptions adcDiffSelect_25: IO324 ADC Setup/adcDiffSelect_25
      mask TypeOptions adcGain_26: IO324 ADC Setup/adcGain_26
      mask TypeOptions adcActiv_26: IO324 ADC Setup/adcActiv_26
      mask TypeOptions adcDiffSelect_26: IO324 ADC Setup/adcDiffSelect_26
      mask TypeOptions adcGain_27: IO324 ADC Setup/adcGain_27
      mask TypeOptions adcActiv_27: IO324 ADC Setup/adcActiv_27
      mask TypeOptions adcDiffSelect_27: IO324 ADC Setup/adcDiffSelect_27
      mask TypeOptions adcGain_28: IO324 ADC Setup/adcGain_28
      mask TypeOptions adcActiv_28: IO324 ADC Setup/adcActiv_28
      mask TypeOptions adcDiffSelect_28: IO324 ADC Setup/adcDiffSelect_28
      mask TypeOptions adcGain_29: IO324 ADC Setup/adcGain_29
      mask TypeOptions adcActiv_29: IO324 ADC Setup/adcActiv_29
      mask TypeOptions adcDiffSelect_29: IO324 ADC Setup/adcDiffSelect_29
      mask TypeOptions adcGain_30: IO324 ADC Setup/adcGain_30
      mask TypeOptions adcActiv_30: IO324 ADC Setup/adcActiv_30
      mask TypeOptions adcDiffSelect_30: IO324 ADC Setup/adcDiffSelect_30
      mask TypeOptions adcGain_31: IO324 ADC Setup/adcGain_31
      mask TypeOptions adcActiv_31: IO324 ADC Setup/adcActiv_31
      mask TypeOptions adcDiffSelect_31: IO324 ADC Setup/adcDiffSelect_31
      mask TypeOptions adcGain_32: IO324 ADC Setup/adcGain_32
      mask TypeOptions adcActiv_32: IO324 ADC Setup/adcActiv_32
      mask TypeOptions adcDiffSelect_32: IO324 ADC Setup/adcDiffSelect_32
      mask TypeOptions dacGain_1: IO324 DAC Setup/dacGain_1
      mask TypeOptions dacActiv_1: IO324 DAC Setup/dacActiv_1
      mask TypeOptions dacGain_2: IO324 DAC Setup/dacGain_2
      mask TypeOptions dacActiv_2: IO324 DAC Setup/dacActiv_2
      mask TypeOptions dacGain_3: IO324 DAC Setup/dacGain_3
      mask TypeOptions dacActiv_3: IO324 DAC Setup/dacActiv_3
      mask TypeOptions dacGain_4: IO324 DAC Setup/dacGain_4
      mask TypeOptions dacActiv_4: IO324 DAC Setup/dacActiv_4
      mask TypeOptions dacGain_5: IO324 DAC Setup/dacGain_5
      mask TypeOptions dacActiv_5: IO324 DAC Setup/dacActiv_5
      mask TypeOptions dacGain_6: IO324 DAC Setup/dacGain_6
      mask TypeOptions dacActiv_6: IO324 DAC Setup/dacActiv_6
      mask TypeOptions dacGain_7: IO324 DAC Setup/dacGain_7
      mask TypeOptions dacActiv_7: IO324 DAC Setup/dacActiv_7
      mask TypeOptions dacGain_8: IO324 DAC Setup/dacGain_8
      mask TypeOptions dacActiv_8: IO324 DAC Setup/dacActiv_8
      mask TypeOptions fpga_sync_mode: IO3xx Setup/fpga_sync_mode
      mask TypeOptions reset_mode: IO3xx Setup/reset_mode
      mask TypeOptions reset_mode_stop: IO3xx Setup/reset_mode_stop
      mask DialogControl ADC Prompt: ADC
      mask DialogControl adcGrp_1 Prompt: Ch 01 to 08
      mask DialogControl adcGrp_2 Prompt: CH 09 to 16
      mask DialogControl adcGrp_3 Prompt: Ch 17 to 24
      mask DialogControl adcGrp_4 Prompt: Ch 25 to 32
      mask DialogControl DAC Prompt: DAC
      mask DialogControl dacGrp_1 Prompt: Ch 01 to 08
      mask Display:
      | SetupBlkPath = sghdlc.model.findSystem(gcb, 'LookUnderMasks', 'all', 'FollowLinks', 'on', 'regexp', 'on', 'Name', 'IO3(\d|x){2}\s+Setup' );
      | SetupBlkPath = SetupBlkPath{1};
      | TS = get_param(SetupBlkPath,'timestamp_mcs');
      | disp(sprintf('Speedgoat IO324-200k\nFPGA I/O Module\n\nTimestamp\n%s\n\nReference Design\nVersion 2.3\n\nMATLAB R2022b\n\nPCIe Link Width: X4\nTiming Severity: error\nRear Plugin: None\nVerifier: off\nVerifier: JTAG\n', TS))
  IO334_FPGA : Subsystem  mask(Speedgoat IO334-325k Interface Block){module_id=1, slot=-1, ts=-1, OutputRange=Auto (same as ADC), fpga_sync_mode=on, reset_mode=on, reset_mode_stop=on, FpgaFreq=100}
      mask prompts: module_id "FPGA Module Identifier:"; slot "PCI slot (-1: autosearch):"; ts "Sample time:"; OutputRange "DAC Voltage Range:"; fpga_sync_mode "Run FPGA only when target application runs"; reset_mode "Reset FPGA states on start"; reset_mode_stop "Reset FPGA states on stop"; FpgaFreq "FPGA Frequency [MHz]"
      mask help: Simulink Real-Time Interface Block for Speedgoat IO334-325k.
      mask init:
      | hdlslrt.backend.mfpgaparameters;
      mask Help: eval('speedgoatdoc_hdlc')
      mask TypeOptions OutputRange: IO334 DAC Setup/OutputRange
      mask TypeOptions fpga_sync_mode: IO3xx Setup/fpga_sync_mode
      mask TypeOptions reset_mode: IO3xx Setup/reset_mode
      mask TypeOptions reset_mode_stop: IO3xx Setup/reset_mode_stop
      mask DialogControl AnalogOutput Prompt: Analog Output
      mask Display:
      | SetupBlkPath = sghdlc.model.findSystem(gcb, 'LookUnderMasks', 'all', 'FollowLinks', 'on', 'regexp', 'on', 'Name', 'IO3(\d|x){2}\s+Setup' );
      | SetupBlkPath = SetupBlkPath{1};
      | TS = get_param(SetupBlkPath,'timestamp_mcs');
      | disp(sprintf('Speedgoat IO334-325k\nFPGA I/O Module\n\nTimestamp\n%s\n\nReference Design\nVersion 2.3\n\nMATLAB R2022b\n\nPCIe Link Width: X4\nTiming Severity: error\nRear Plugin: None\nAurora Mode: None\nAurora Crc: true\nAurora Byteswap: true\nVerifier: off\nVerifier: JTAG\n', TS))
  IO397_FPGA : Subsystem  mask(Speedgoat IO397-50k Interface Block){module_id=1, slot=-1, ts=-1, range1=+-10 V, range2=+-10 V, range3=+-10 V, range4=+-10 V, span=+-10 V, fpga_sync_mode=on, reset_mode=on, reset_mode_stop=on, FpgaFreq=100}
      mask prompts: module_id "FPGA Module Identifier:"; slot "PCI slot (-1: autosearch):"; ts "Sample time:"; range1 "Range ADC Channel 1"; range2 "Range ADC Channel 2"; range3 "Range ADC Channel 3"; range4 "Range ADC Channel 4"; span "DAC Voltage Span:"; fpga_sync_mode "Run FPGA only when target application runs"; reset_mode "Reset FPGA states on start"; reset_mode_stop "Reset FPGA states on stop"; FpgaFreq "FPGA Frequency [MHz]"
      mask help: Simulink Real-Time Interface Block for Speedgoat IO397-50k.
      mask init:
      | hdlslrt.backend.mfpgaparameters;
      mask Help: eval('speedgoatdoc_hdlc')
      mask TypeOptions range1: IO397 ADC Setup/range1
      mask TypeOptions range2: IO397 ADC Setup/range2
      mask TypeOptions range3: IO397 ADC Setup/range3
      mask TypeOptions range4: IO397 ADC Setup/range4
      mask TypeOptions span: IO397 DAC Setup/span
      mask TypeOptions fpga_sync_mode: IO3xx Setup/fpga_sync_mode
      mask TypeOptions reset_mode: IO3xx Setup/reset_mode
      mask TypeOptions reset_mode_stop: IO3xx Setup/reset_mode_stop
      mask DialogControl AnalogInput Prompt: Analog Input
      mask DialogControl AnalogOutput Prompt: Analog Output
      mask Display:
      | SetupBlkPath = sghdlc.model.findSystem(gcb, 'LookUnderMasks', 'all', 'FollowLinks', 'on', 'regexp', 'on', 'Name', 'IO3(\d|x){2}\s+Setup' );
      | SetupBlkPath = SetupBlkPath{1};
      | TS = get_param(SetupBlkPath,'timestamp_mcs');
      | disp(sprintf('Speedgoat IO397-50k\nFPGA I/O Module\n\nTimestamp\n%s\n\nReference Design\nVersion 2.3\n\nMATLAB R2022b\n\nPCIe Link Width: X1\nTiming Severity: error\nVerifier: off\nVerifier: JTAG\n', TS))

== system SG_library/Source elements/ADC trigger ==
  ticks : Inport
  Decrement Stored Integer : simulink/Additional Math & Discrete/Additional Math: Increment - Decrement/Decrement Stored Integer
  HDL Counter : hdlsllib/Sources/HDL Counter  CountType=Free running  CountInit=uint32(0)  CountStep=uint32(1)  CountMax=25  CountFromType=Initial value  CountFrom=uint32(0)  CountResetPort=on  CountLoadPort=off  CountEnbPort=off  CountDirPort=off  CountHitOutputPort=off  CountDataType=Unsigned  CountWordLen=32  CountFracLen=0  CountSampTime=1
  Relational Operator1 : RelationalOperator  Operator=<=  OutDataTypeStr=boolean  RndMeth=Simplest  InputSameDT=off
  Unit Delay : UnitDelay  SampleTime=-1  HasFrameUpgradeWarning=on
  trig : Outport  VectorParamsAs1DForOutWhenUnconnected=off
  wires:
  HDL Counter/1 -> Relational Operator1/2
  Relational Operator1/1 -> HDL Counter/1, Unit Delay/1
  ticks/1 -> Decrement Stored Integer/1
  Decrement Stored Integer/1 -> Relational Operator1/1
  Unit Delay/1 -> trig/1

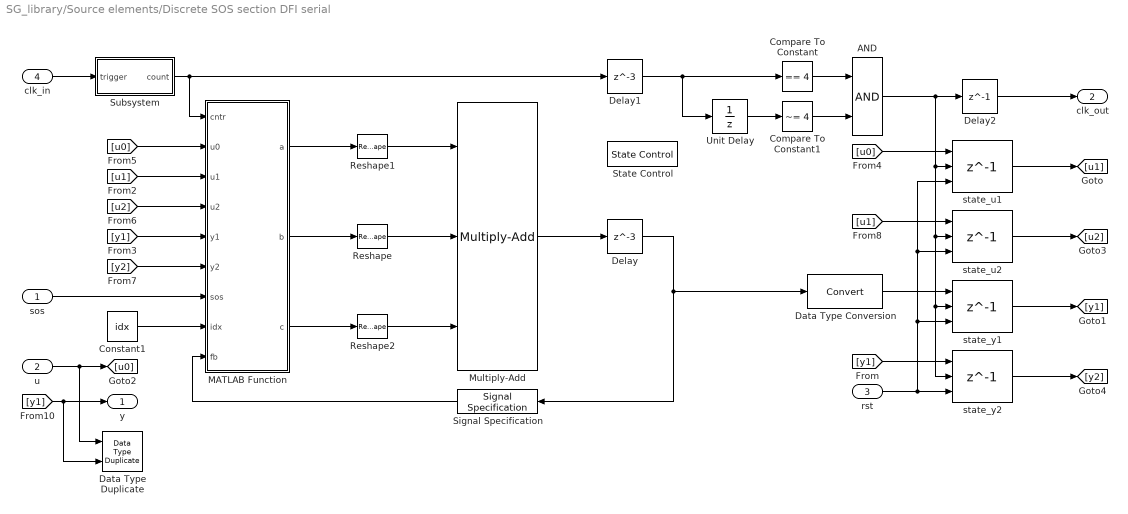
== system SG_library/Source elements/Discrete SOS section DFI serial ==
  sos : Inport
  u : Inport  Port=2
  rst : Inport  Port=3
  clk_in : Inport  Port=4
  AND : Logic  AllPortsSameDT=off  OutDataTypeStr=boolean
  Compare To Constant : simulink/Logic and Bit Operations/Compare To Constant  relop===  const=4  OutDataTypeStr=boolean
  Compare To Constant1 : simulink/Logic and Bit Operations/Compare To Constant  relop=~=  const=4  OutDataTypeStr=boolean
  Constant1 : Constant  Value=idx  OutDataTypeStr=uint8  SampleTime=-1
  Data Type Duplicate : DataTypeDuplicate
  Data Type Conversion : DataTypeConversion  SaturateOnIntegerOverflow=off  RndMeth=Floor
  Delay : Delay  DelayLength=3
  Delay1 : Delay  DelayLength=3
  Delay2 : Delay  DelayLength=1
  MATLAB Function : MATLAB Function  TreatAsAtomicUnit=on
  Multiply-Add : hdlsllib/HDL Operations/Multiply-Add  Function=c+(a.*b)  datatype=Inherit: Inherit via back propagation  RndMeth=Simplest  DoSatur=on  FMA=off
  Reshape : Reshape
  Reshape1 : Reshape
  Reshape2 : Reshape
  Signal Specification : SignalSpecification  OutDataTypeStr=fixdt(1,80,52)
  State Control : StateControl  StateControl=Synchronous
  Subsystem : Subsystem
  Unit Delay : UnitDelay  SampleTime=-1  HasFrameUpgradeWarning=on
  state_u1 : Delay  DelayLength=1  ExternalReset=Level hold  ShowEnablePort=on
      settings: InputPortMap=u0,e6,r5
  state_u2 : Delay  DelayLength=1  ExternalReset=Level hold  ShowEnablePort=on
      settings: InputPortMap=u0,e6,r5
  state_y1 : Delay  DelayLength=1  ExternalReset=Level hold  ShowEnablePort=on
      settings: InputPortMap=u0,e6,r5
  state_y2 : Delay  DelayLength=1  ExternalReset=Level hold  ShowEnablePort=on
      settings: InputPortMap=u0,e6,r5
  y : Outport  InitialOutput=0  VectorParamsAs1DForOutWhenUnconnected=off
  clk_out : Outport  Port=2
  wires:
  Delay2/1 -> clk_out/1
  clk_in/1 -> Subsystem/1(trigger)
  Multiply-Add/1 -> Delay/1
  Delay/1 -> Signal Specification/1, Data Type Conversion/1
  Subsystem/1(count) -> MATLAB Function/1(cntr), Delay1/1
  Compare To Constant/1 -> AND/1
  Delay1/1 -> Unit Delay/1, Compare To Constant/1
  Unit Delay/1 -> Compare To Constant1/1
  AND/1 -> state_y2/2, state_y1/2, state_u2/2, state_u1/2, Delay2/1
  u/1 -> Data Type Duplicate/1, [u0]
  [y1] -> Data Type Duplicate/2, y/1
  Compare To Constant1/1 -> AND/2
  [u0] -> state_u1/1
  [u1] -> state_u2/1
  [y1] -> state_y2/1
  [u0] -> MATLAB Function/2(u0)
  [u1] -> MATLAB Function/3(u1)
  [u2] -> MATLAB Function/4(u2)
  [y1] -> MATLAB Function/5(y1)
  [y2] -> MATLAB Function/6(y2)
  sos/1 -> MATLAB Function/7(sos)
  Constant1/1 -> MATLAB Function/8(idx)
  Signal Specification/1 -> MATLAB Function/9(fb)
  MATLAB Function/1(a) -> Reshape1/1
  MATLAB Function/2(b) -> Reshape/1
  MATLAB Function/3(c) -> Reshape2/1
  Data Type Conversion/1 -> state_y1/1
  rst/1 -> state_y2/3, state_y1/3, state_u2/3, state_u1/3
  state_u1/1 -> [u1]
  state_u2/1 -> [u2]
  state_y1/1 -> [y1]
  state_y2/1 -> [y2]
  Reshape/1 -> Multiply-Add/2
  Reshape1/1 -> Multiply-Add/1
  Reshape2/1 -> Multiply-Add/3

== system SG_library/Source elements/Discrete SOS serial ==
  u : Inport
  sos : Inport  Port=2
  reset : Inport  Port=3
  clk_in : Inport  Port=4
  Delay : Delay  DelayLength=1  ShowEnablePort=on
      settings: InputPortMap=u0,e6
  Delay1 : Delay  DelayLength=1
  Discrete SOS section DFI serial : $bdroot/Source elements/Discrete SOS section DFI serial  idx=1  OutDataTypeStr=fixdt(1,80,52)
      settings: LibrarySourceBlock=|
      | SG_library/Source elements/Discrete SOS
      | section DF1
  Discrete SOS section DFI serial1 : $bdroot/Source elements/Discrete SOS section DFI serial  idx=2  OutDataTypeStr=fixdt(1,80,52)
      settings: LibrarySourceBlock=|
      | SG_library/Source elements/Discrete SOS
      | section DF1
  Discrete SOS section DFI serial2 : $bdroot/Source elements/Discrete SOS section DFI serial  idx=3  OutDataTypeStr=fixdt(1,80,52)
      settings: LibrarySourceBlock=|
      | SG_library/Source elements/Discrete SOS
      | section DF1
  Discrete SOS section DFI serial3 : $bdroot/Source elements/Discrete SOS section DFI serial  idx=4  OutDataTypeStr=fixdt(1,80,52)
      settings: LibrarySourceBlock=|
      | SG_library/Source elements/Discrete SOS
      | section DF1
  State Control : StateControl  StateControl=Synchronous
  y : Outport  InitialOutput=0  VectorParamsAs1DForOutWhenUnconnected=off
  clk_out : Outport  Port=2
  wires:
  clk_in/1 -> Delay/2, Delay1/1
  u/1 -> Delay/1
  reset/1 -> Discrete SOS section DFI serial/3, Discrete SOS section DFI serial1/3, Discrete SOS section DFI serial2/3, Discrete SOS section DFI serial3/3
  Delay/1 -> Discrete SOS section DFI serial/2
  Delay1/1 -> Discrete SOS section DFI serial/4
  Discrete SOS section DFI serial2/1 -> Discrete SOS section DFI serial3/2
  Discrete SOS section DFI serial2/2 -> Discrete SOS section DFI serial3/4
  Discrete SOS section DFI serial1/1 -> Discrete SOS section DFI serial2/2
  Discrete SOS section DFI serial1/2 -> Discrete SOS section DFI serial2/4
  Discrete SOS section DFI serial/1 -> Discrete SOS section DFI serial1/2
  Discrete SOS section DFI serial/2 -> Discrete SOS section DFI serial1/4
  Discrete SOS section DFI serial3/1 -> y/1
  Discrete SOS section DFI serial3/2 -> clk_out/1
  sos/1 -> Discrete SOS section DFI serial3/1, Discrete SOS section DFI serial2/1, Discrete SOS section DFI serial1/1, Discrete SOS section DFI serial/1

== system SG_library/Source elements/Generator ==
  start : Inport
  cancel : Inport  Port=2
  on : Inport  Port=3
  Constant : Constant  Value=duration  SampleTime=-1
  Constant1 : Constant  Value=gen_type  OutDataTypeStr=Enum: GeneratorType  SampleTime=-1
  OR : Logic  Operator=OR  AllPortsSameDT=off  OutDataTypeStr=boolean
  Signal Specification : SignalSpecification  SampleTime=ts
  Triggered Pulse : $bdroot/Source elements/Triggered Pulse
  Weighted Sample Time : SampleTimeMath  TsampMathOp=/
  gen : Subsystem  TreatAsAtomicUnit=on
  rms : Gain  Gain=rms
  signal : Outport
  enabled : Outport  Port=2
  wires:
  Triggered Pulse/1 -> Signal Specification/1, OR/1
  OR/1 -> gen/Enable
  gen/1(signal) -> rms/1
  rms/1 -> signal/1
  Signal Specification/1 -> enabled/1
  start/1 -> Triggered Pulse/1
  cancel/1 -> Triggered Pulse/2
  on/1 -> OR/2
  Constant/1 -> Weighted Sample Time/1
  Weighted Sample Time/1 -> Triggered Pulse/3
  Constant1/1 -> gen/1(type)

== system SG_library/Source elements/Linear Chirp ==
  MATLAB Function : MATLAB Function  TreatAsAtomicUnit=on
  Probe Sample Time : Probe  ProbeWidth=off  ProbeComplexSignal=off
  Selector : Selector  IndexOptions=Index vector (dialog)  Indices=1  OutputSizes=1
  Signal Specification : SignalSpecification  SampleTime=ts
  Subsystem : Subsystem
  y : Outport
  wires:
  Subsystem/1(cntr) -> Signal Specification/1, Probe Sample Time/1
  MATLAB Function/1(y) -> y/1
  Probe Sample Time/1 -> Selector/1
  Signal Specification/1 -> MATLAB Function/1(cnt)
  Selector/1 -> MATLAB Function/2(ts)

== system SG_library/Source elements/Logarithmic Chirp ==
  MATLAB Function : MATLAB Function  TreatAsAtomicUnit=on
  Probe Sample Time : Probe  ProbeWidth=off  ProbeComplexSignal=off
  Selector : Selector  IndexOptions=Index vector (dialog)  Indices=1  OutputSizes=1
  Signal Specification : SignalSpecification  SampleTime=ts
  Subsystem : Subsystem
  y : Outport
  wires:
  Subsystem/1(cntr) -> Signal Specification/1, Probe Sample Time/1
  MATLAB Function/1(y) -> y/1
  Probe Sample Time/1 -> Selector/1
  Signal Specification/1 -> MATLAB Function/1(cnt)
  Selector/1 -> MATLAB Function/2(ts)

== system SG_library/Source elements/Random source ==
  Bias : Bias  Bias=mean  SaturateOnIntegerOverflow=off
  Discrete Filter : DiscreteFilter  Numerator=[0.5 0.5]  Denominator=[1 0.1]  InputProcessing=Columns as channels (frame based)  FilterStructure=Direct form II transposed  a0EqualsOne=on
  Gain : Gain  Gain=stdev
  Random Number : RandomNumber  Seed=seed  SampleTime=SampleTime
  x : Outport  VectorParamsAs1DForOutWhenUnconnected=off
  wires:
  Random Number/1 -> Gain/1
  Discrete Filter/1 -> x/1
  Gain/1 -> Bias/1
  Bias/1 -> Discrete Filter/1

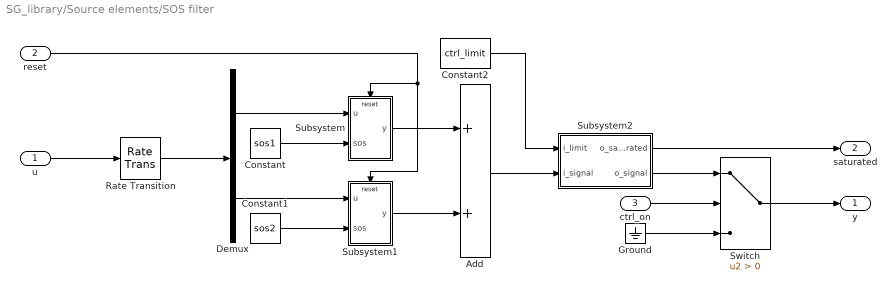
== system SG_library/Source elements/SOS filter ==
  u : Inport
  reset : Inport  Port=2
  ctrl_on : Inport  Port=3
  Add : Sum  OutDataTypeStr=double
  Constant : Constant  Value=sos1  SampleTime=-1
  Constant1 : Constant  Value=sos2  SampleTime=-1
  Constant2 : Constant  Value=ctrl_limit  SampleTime=-1
  Demux : Demux  Outputs=2
  Ground : Ground
  Rate Transition : RateTransition  OutPortSampleTime=ts
  Subsystem : Subsystem
  Subsystem1 : Subsystem
  Subsystem2 : Subsystem
  Switch : Switch  Criteria=u2 > Threshold  SaturateOnIntegerOverflow=off  InputSameDT=off
  y : Outport  VectorParamsAs1DForOutWhenUnconnected=off
  saturated : Outport  Port=2
  wires:
  Subsystem2/2(o_signal) -> Switch/1
  ctrl_on/1 -> Switch/2
  Switch/1 -> y/1
  Ground/1 -> Switch/3
  Add/1 -> Subsystem2/2(i_signal)
  u/1 -> Rate Transition/1
  Constant1/1 -> Subsystem1/2(sos)
  Subsystem/1(y) -> Add/1
  Constant/1 -> Subsystem/2(sos)
  Demux/1 -> Subsystem/1(u)
  Demux/2 -> Subsystem1/1(u)
  Subsystem1/1(y) -> Add/2
  reset/1 -> Subsystem1/Reset, Subsystem/Reset
  Rate Transition/1 -> Demux/1
  Subsystem2/1(o_saturated) -> saturated/1
  Constant2/1 -> Subsystem2/1(i_limit)
